simulink model "VGrowth"  (R2018b)
settings: Solver=VariableStepAuto  StartTime=0.0  StopTime=50  RelTol=1e-3
libraries: simulink x1
settings Model: Creator=Magneto  LastModifiedBy=Magneto

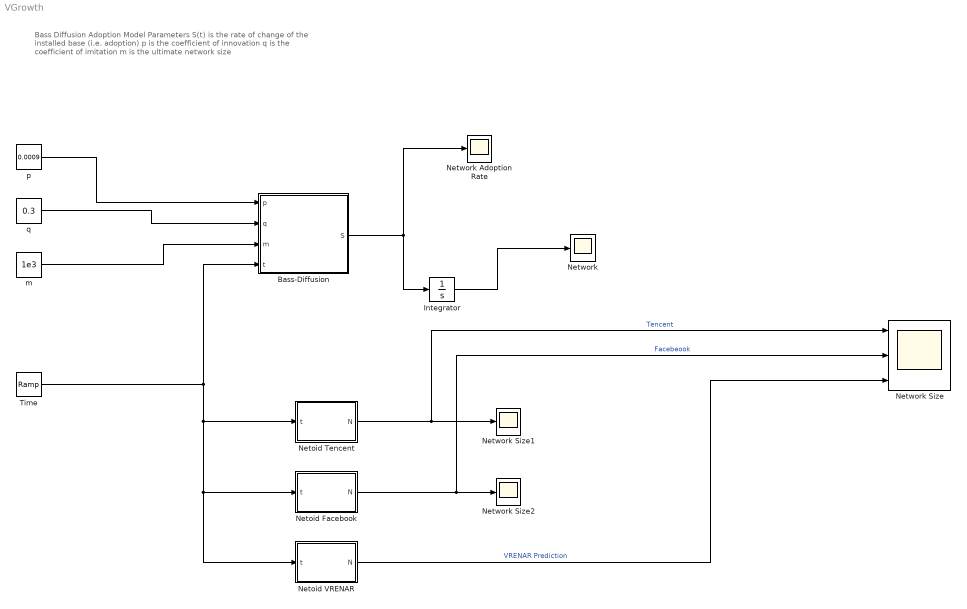
== system VGrowth ==
  note: Bass Diffusion Adoption Model Parameters
      | S(t) is the rate of change of the installed base (i.e. adoption)
      | p is the coefficient of innovation
      | q is the coefficient of imitation
      | m is the ultimate network size
  Bass-Diffusion : MATLAB Function  TreatAsAtomicUnit=on
  Integrator : Integrator
  Netoid Facebook : MATLAB Function  TreatAsAtomicUnit=on
  Netoid Tencent : MATLAB Function  TreatAsAtomicUnit=on
  Netoid VRENAR : MATLAB Function  TreatAsAtomicUnit=on
  Network : Scope
  Network Adoption Rate : Scope
  Network Size : Scope  NumInputPorts=3
  Network Size1 : Scope
  Network Size2 : Scope
  Time : simulink/Sources/Ramp  slope=1  start=0  InitialOutput=0
  m : Constant  Value=1e3
  p : Constant  Value=0.0009
  q : Constant  Value=0.3
  wires:
  p/1 -> Bass-Diffusion/1(p)
  q/1 -> Bass-Diffusion/2(q)
  m/1 -> Bass-Diffusion/3(m)
  Bass-Diffusion/1(S) -> Network Adoption Rate/1, Integrator/1
  Time/1 -> Bass-Diffusion/4(t), Netoid VRENAR/1(t), Netoid Facebook/1(t), Netoid Tencent/1(t)
  Netoid Facebook/1(N) -> Network Size/2, Network Size2/1  "Facebeook"
  Netoid Tencent/1(N) -> Network Size/1, Network Size1/1  "Tencent"
  Integrator/1 -> Network/1
  Netoid VRENAR/1(N) -> Network Size/3  "VRENAR Prediction"

== matlab function VGrowth/Netoid Tencent ==
  data: t input; N output
function N = fcn(t)

N = 2.61e9/(1+exp(-0.3*(t-15)));

== matlab function VGrowth/Bass-Diffusion ==
  data: p input; S output; q input; m input; t input
function S = fcn(p,q,m,t)

S = m*(((p+q)^2)/p)*(exp(-(p+q)*t)/(1+((q/p)*exp(-(p+q)*t)))^2);

== matlab function VGrowth/Netoid Facebook ==
  data: t input; N output
function N = fcn(t)

N = 1.45e9/(1+exp(-0.77*(t-10)));

== matlab function VGrowth/Netoid VRENAR ==
  data: t input; N output
function N = fcn(t)

N = 1.45e9/(1+exp(-0.77*(t-10)));
